simulink model "HW10_18EE30021_22Mar"  (R2020b)
settings: Solver=ode23t  StartTime=0.0  StopTime=1e-7  RelTol=1e-3
libraries: powerlib x20
settings Model: Creator=user  LastModifiedBy=Pratyush Jaiswal
settings DataIOCC: ReturnWorkspaceOutputs=off
settings DebuggingCC: ArithmeticOperatorsInVariantConditions=warning
settings SFSimCC: CustomCodeUndefinedFunction=UseInterfaceOnly

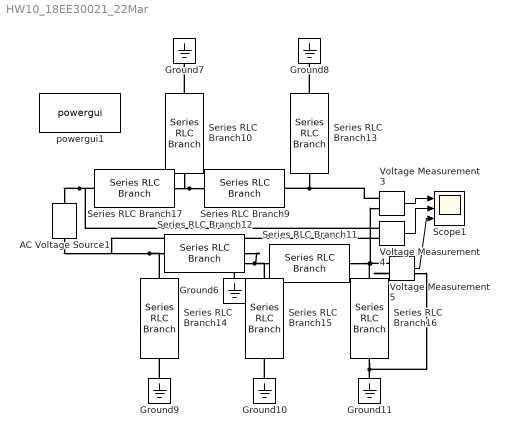
== system HW10_18EE30021_22Mar ==
  AC Voltage Source1 : powerlib/Electrical Sources/AC Voltage Source  Amplitude=5  Phase=0  Frequency=1e9  SampleTime=0  Measurements=None  BusType=swing  Pref=10e3  Qref=0  Qmin=-inf  Qmax=+inf
  Ground{6..11} (6 alike) : powerlib/Elements/Ground  LConnTagsString=a
  Scope1 : Scope  NumInputPorts=3
  Series RLC Branch{10,13..16} (5 alike) : powerlib/Elements/Series RLC Branch  LConnTagsString=__new0  RConnTagsString=__new0  BranchType=C  Resistance=1  Inductance=1e-10  SetiL0=off  InitialCurrent=0  Capacitance=1e-12  Setx0=off  InitialVoltage=0  Measurements=None
  Series RLC Branch11 : powerlib/Elements/Series RLC Branch  LConnTagsString=__new0  RConnTagsString=__new0  BranchType=L  Resistance=1  Inductance=1e-10  SetiL0=off  InitialCurrent=0  Capacitance=1e-6  Setx0=off  InitialVoltage=0  Measurements=None
  Series RLC Branch12 : powerlib/Elements/Series RLC Branch  LConnTagsString=__new0  RConnTagsString=__new0  BranchType=L  Resistance=1  Inductance=1e-10  SetiL0=off  InitialCurrent=0  Capacitance=1e-6  Setx0=off  InitialVoltage=0  Measurements=None
  Series RLC Branch17 : powerlib/Elements/Series RLC Branch  LConnTagsString=__new0  RConnTagsString=__new0  BranchType=R  Resistance=50  Inductance=1e-3  SetiL0=off  InitialCurrent=0  Capacitance=1e-6  Setx0=off  InitialVoltage=0  Measurements=None
  Series RLC Branch9 : powerlib/Elements/Series RLC Branch  LConnTagsString=__new0  RConnTagsString=__new0  BranchType=L  Resistance=1  Inductance=1e-10  SetiL0=off  InitialCurrent=0  Capacitance=1e-6  Setx0=off  InitialVoltage=0  Measurements=None
  Voltage Measurement3 : powerlib/Measurements/Voltage Measurement  PhasorSimulation=off  OutputType=Complex  PSBequivalent=0
  Voltage Measurement4 : powerlib/Measurements/Voltage Measurement  PhasorSimulation=off  OutputType=Complex  PSBequivalent=0
  Voltage Measurement5 : powerlib/Measurements/Voltage Measurement  PhasorSimulation=off  OutputType=Complex  PSBequivalent=0
  powergui1 : powerlib/powergui  Priority=1  SimulationMode=Continuous  SampleTime=50e-6  frequency=60  Iterations=50  frequencyindice=1000000000  Pbase=100e6  ErrMax=1e-4  UnitsV=kV  UnitsW=MW  buscounter=0  FunctionMessages=off  echomessages=off  EnableUseOfTLC=off  CurrentSourceSwitches=off  DisableSnubberDevices=off  DisableRonSwitches=off  DisableVfSwitches=off  DisplayEquations=off  AutomaticDiscreteSolvers=off  SolverType=Tustin/Backward Euler (TBE)  Interpol=off  ExternalGateDelay=off  methode=off  Ts=100  x0status=blocks  SPID=on  SwTol=0  HookPort=off  NonlinearTolerance=1e-4  nMaxIteration=100  ContinueOnMaxIteration=off  RestoreLinks=warning  ResistiveCurrentMeasurement=off  Frange=[0:2:500]  Ylog=off  Xlog=on  ShowGrid=off  save=off  variable=ZData  structure=0  ZoomFFT=off  StartTime=0.0  cycles=1  DisplayStyle=1  fundamental=60  FreqAxis=off  MaxFrequency=1000  frequencyindicesteady=1  RmsSteady=1  display=off
  wires:
  Voltage Measurement5/1 -> Scope1/3
  Voltage Measurement4/1 -> Scope1/2
  Voltage Measurement3/1 -> Scope1/1
  connections:
  Series RLC Branch11/RConn1 -- Series RLC Branch16/LConn1 -- Voltage Measurement5/LConn1 -- Voltage Measurement3/LConn2
  Voltage Measurement3/LConn1 -- Series RLC Branch9/RConn1 -- Series RLC Branch13/LConn1
  Ground6/LConn1 -- Series RLC Branch11/LConn1 -- Series RLC Branch12/RConn1 -- Series RLC Branch15/LConn1
  Series RLC Branch14/LConn1 -- Series RLC Branch12/LConn1 -- AC Voltage Source1/LConn1 -- Voltage Measurement4/LConn2
  Voltage Measurement5/LConn2 -- Series RLC Branch16/RConn1 -- Ground11/LConn1
  Series RLC Branch10/LConn1 -- Series RLC Branch9/LConn1 -- Series RLC Branch17/RConn1
  Series RLC Branch17/LConn1 -- AC Voltage Source1/RConn1 -- Voltage Measurement4/LConn1
  Series RLC Branch13/RConn1 -- Ground8/LConn1
  Ground9/LConn1 -- Series RLC Branch14/RConn1
  Series RLC Branch10/RConn1 -- Ground7/LConn1
  Ground10/LConn1 -- Series RLC Branch15/RConn1
